simulink model "gm_uz_endat_interface_2025b"  (R2025b)
settings: Solver=FixedStepDiscrete  StartTime=0.0  StopTime=1.3e-3  RelTol=1e-3
undefined symbols (not defined in the file or in its folder): binary_or_gray, bit_sum, delay_first_clk_on_off, endat_clk_divider, endat_encoder_bit_width_multi_turn, endat_encoder_bit_width_single_turn, endat_encoder_number_of_CRC_bits, f_ADC, f_clock, PLL, t_ADC, t_clock, XData
libraries: hdlmdlgenlib x123, simulink x35, hdlsllib x29, simulink_extras x13
(part 4 of 4)

== system gm_uz_endat_interface_2025b/uz_endat_interface/position_to_speed_pll/Sine HDL Optimized/sincos hdl/cos_hdl ==
  note: (C) 2016 Mathworks, Inc
  In1 : Inport  OutDataTypeStr=fixdt(1, 27, 20)  SampleTime=1e-08
  1st or 4th Quad : Logic  Operator=OR  AllPortsSameDT=off  OutDataTypeStr=boolean  SampleTime=1e-08
  Amp25 : Sum  Inputs=+-  OutDataTypeStr=fixdt(1, 28, 27)  AccumDataTypeStr=fixdt(1, 28, 27)  SampleTime=1e-08
  Amp75 : Sum  Inputs=+-  OutDataTypeStr=fixdt(1, 28, 27)  AccumDataTypeStr=fixdt(1, 28, 27)  SampleTime=1e-08
  CastU16En1 : DataTypeConversion  OutDataTypeStr=fixdt(0, 10, 0)  ConvertRealWorld=Stored Integer (SI)  SampleTime=1e-08  SaturateOnIntegerOverflow=off  RndMeth=Floor
  CastU16En2 : DataTypeConversion  OutDataTypeStr=fixdt(0, 10, 0)  ConvertRealWorld=Stored Integer (SI)  SampleTime=1e-08  RndMeth=Floor
  CastU16En3 : DataTypeConversion  OutDataTypeStr=fixdt(0, 11, 0)  SampleTime=1e-08  SaturateOnIntegerOverflow=off  RndMeth=Floor
  GTEp75 : RelationalOperator  OutDataTypeStr=boolean  SampleTime=1e-08  InputSameDT=off
  LTEp25 : RelationalOperator  Operator=<=  OutDataTypeStr=boolean  SampleTime=1e-08  InputSameDT=off
  LTEp50 : RelationalOperator  Operator=<=  OutDataTypeStr=boolean  SampleTime=1e-08  InputSameDT=off
  Look-Up Table : Lookup_n-D  NumberOfTableDimensions=1  LookupTableObject=''  BreakpointsSpecification=Even spacing  BreakpointsForDimension1=XData  BreakpointsForDimension1FirstPoint=fi(0,0,InputWordLength,0)  BreakpointsForDimension1Spacing=fi(1,0,InputWordLength,0)  IndexSearchMethod=Evenly spaced points  Table=fi(YData,0, TableWordLength, TableFracLength)  TableDataTypeStr=fixdt(0, TableWordLength, TableFracLength)  InterpMethod=Flat  ExtrapMethod=Clip  OutDataTypeStr=fixdt(1,OutputWordLength,OutputFracLength)  LockScale=on
  Negate : UnaryMinus  SampleTime=1e-08
  Point25 : Constant  Value=0.25  OutDataTypeStr=fixdt(0, 27, 27)  SampleTime=1e-08
  Point50 : Constant  Value=0.5  OutDataTypeStr=fixdt(0, 27, 27)  SampleTime=1e-08
  Point75 : Constant  Value=0.75  OutDataTypeStr=fixdt(0, 27, 27)  SampleTime=1e-08
  Positive : DataTypeConversion  OutDataTypeStr=fixdt('sfix27_En20')
  QuadHandle1a : Switch  Criteria=u2 ~= 0  Threshold="fi(0,0,1,0,\"hex\",\"0\")"  OutDataTypeStr=fixdt(1, 28, 27)  SampleTime=1e-08  SaturateOnIntegerOverflow=off  InputSameDT=off
  QuadHandle1b : Switch  Criteria=u2 ~= 0  Threshold="fi(0,0,1,0,\"hex\",\"0\")"  OutDataTypeStr=fixdt(1, 28, 27)  SampleTime=1e-08  SaturateOnIntegerOverflow=off  InputSameDT=off
  QuadHandle2 : Switch  Criteria=u2 ~= 0  Threshold="fi(0,0,1,0,\"hex\",\"0\")"  OutDataTypeStr=fixdt(0, 10, 10)  SampleTime=1e-08  InputSameDT=off
  RAMDelayBalance : hdlmdlgenlib/Buffer
  Saturation : Saturate  UpperLimit="fi(0,0,10,0,\"hex\",\"0ff\")"  LowerLimit="fi(0,0,10,0,\"hex\",\"000\")"  SampleTime=1e-08  OutDataTypeStr=fixdt(0, 10, 0)
  SignCorrected : Switch  Criteria=u2 ~= 0  Threshold="fi(0,0,8,0,\"hex\",\"00\")"  OutDataTypeStr=fixdt(1, 27, 20)  SampleTime=1e-08  SaturateOnIntegerOverflow=off  InputSameDT=off
  Switch : Switch  Criteria=u2 ~= 0  Threshold="fi(0,0,1,0,\"hex\",\"0\")"  OutDataTypeStr=fixdt(0, 10, 0)  SampleTime=1e-08  SaturateOnIntegerOverflow=off  InputSameDT=off
  dtc : DataTypeConversion  OutDataTypeStr=uint8  ConvertRealWorld=Stored Integer (SI)  SampleTime=1e-08  SaturateOnIntegerOverflow=off  RndMeth=Floor
  insig : DataTypeConversion  OutDataTypeStr=fixdt(0, 10, 10)  SampleTime=1e-08  SaturateOnIntegerOverflow=off  RndMeth=Floor
  p25mA : Sum  Inputs=+-  OutDataTypeStr=fixdt(1, 28, 27)  AccumDataTypeStr=fixdt(1, 28, 27)  SampleTime=1e-08
  p75mA : Sum  Inputs=+-  OutDataTypeStr=fixdt(1, 28, 27)  AccumDataTypeStr=fixdt(1, 28, 27)  SampleTime=1e-08
  pow2switch : Constant  OutDataTypeStr=boolean  SampleTime=1e-08
  x : Outport  SampleTime=1e-08  VectorParamsAs1DForOutWhenUnconnected=off
  wires:
  LTEp25/1 -> 1st or 4th Quad/1, QuadHandle1a/2
  Point50/1 -> LTEp50/2
  In1/1 -> insig/1
  Point25/1 -> p25mA/1, Amp25/2, LTEp25/2
  insig/1 -> LTEp50/1, p25mA/2, GTEp75/1, Amp75/1, LTEp25/1, Amp25/1, p75mA/2
  Point75/1 -> p75mA/1, GTEp75/2, Amp75/2
  p25mA/1 -> QuadHandle1a/1
  GTEp75/1 -> QuadHandle1b/2, 1st or 4th Quad/2
  Amp25/1 -> QuadHandle1a/3
  LTEp50/1 -> QuadHandle2/2
  Amp75/1 -> QuadHandle1b/1
  p75mA/1 -> QuadHandle1b/3
  pow2switch/1 -> Switch/2
  1st or 4th Quad/1 -> dtc/1
  QuadHandle1a/1 -> QuadHandle2/1
  QuadHandle1b/1 -> QuadHandle2/3
  dtc/1 -> RAMDelayBalance/1
  RAMDelayBalance/1 -> SignCorrected/2
  QuadHandle2/1 -> CastU16En1/1
  CastU16En1/1 -> CastU16En3/1
  CastU16En3/1 -> CastU16En2/1
  CastU16En2/1 -> Switch/3, Saturation/1
  Saturation/1 -> Switch/1
  Switch/1 -> Look-Up Table/1
  Look-Up Table/1 -> Positive/1, Negate/1
  Positive/1 -> SignCorrected/1
  Negate/1 -> SignCorrected/3
  SignCorrected/1 -> x/1

== system gm_uz_endat_interface_2025b/uz_endat_interface/position_to_speed_pll/Sine HDL Optimized/sincos hdl/sin_hdl ==
  note: (C) 2016 Mathworks, Inc
  In1 : Inport  OutDataTypeStr=fixdt(1, 27, 20)  SampleTime=1e-08
  Amp50 : Sum  Inputs=+-  OutDataTypeStr=fixdt(1, 28, 27)  AccumDataTypeStr=fixdt(1, 28, 27)  SampleTime=1e-08
  CastU16En2 : DataTypeConversion  OutDataTypeStr=fixdt(0, 10, 0)  ConvertRealWorld=Stored Integer (SI)  SampleTime=1e-08  SaturateOnIntegerOverflow=off  RndMeth=Floor
  CastU16En3 : DataTypeConversion  OutDataTypeStr=fixdt(0, 10, 0)  ConvertRealWorld=Stored Integer (SI)  SampleTime=1e-08  RndMeth=Floor
  CastU16En4 : DataTypeConversion  OutDataTypeStr=fixdt(0, 11, 0)  SampleTime=1e-08  SaturateOnIntegerOverflow=off  RndMeth=Floor
  LTEp25 : RelationalOperator  Operator=<=  OutDataTypeStr=boolean  SampleTime=1e-08  InputSameDT=off
  LTEp50 : RelationalOperator  Operator=<=  OutDataTypeStr=boolean  SampleTime=1e-08  InputSameDT=off
  Look-Up Table : Lookup_n-D  NumberOfTableDimensions=1  LookupTableObject=''  BreakpointsSpecification=Even spacing  BreakpointsForDimension1=XData  BreakpointsForDimension1FirstPoint=fi(0,0,InputWordLength,0)  BreakpointsForDimension1Spacing=fi(1,0,InputWordLength,0)  IndexSearchMethod=Evenly spaced points  Table=fi(YData,0, TableWordLength, TableFracLength)  TableDataTypeStr=fixdt(0, TableWordLength, TableFracLength)  InterpMethod=Flat  ExtrapMethod=Clip  OutDataTypeStr=fixdt(1,OutputWordLength,OutputFracLength)  LockScale=on
  Negate : UnaryMinus  SampleTime=1e-08
  Point25 : Constant  Value=0.25  OutDataTypeStr=fixdt(0, 27, 27)  SampleTime=1e-08
  Point50 : Constant  Value=0.5  OutDataTypeStr=fixdt(0, 27, 27)  SampleTime=1e-08
  Positive : DataTypeConversion  OutDataTypeStr=fixdt('sfix27_En20')
  QuadHandle1 : Switch  Criteria=u2 ~= 0  Threshold="fi(0,0,1,0,\"hex\",\"0\")"  OutDataTypeStr=fixdt(1, 28, 27)  SampleTime=1e-08  SaturateOnIntegerOverflow=off  InputSameDT=off
  QuadHandle2 : Switch  Criteria=u2 ~= 0  Threshold="fi(0,0,1,0,\"hex\",\"0\")"  OutDataTypeStr=fixdt(0, 10, 10)  SampleTime=1e-08  SaturateOnIntegerOverflow=off  InputSameDT=off
  RAMDelayBalance : hdlmdlgenlib/Buffer
  Saturation : Saturate  UpperLimit="fi(0,0,10,0,\"hex\",\"0ff\")"  LowerLimit="fi(0,0,10,0,\"hex\",\"000\")"  SampleTime=1e-08  OutDataTypeStr=fixdt(0, 10, 0)
  SignCorrected : Switch  Criteria=u2 ~= 0  Threshold="fi(0,0,1,0,\"hex\",\"0\")"  OutDataTypeStr=fixdt(1, 27, 20)  SampleTime=1e-08  SaturateOnIntegerOverflow=off  InputSameDT=off
  Switch : Switch  Criteria=u2 ~= 0  Threshold="fi(0,0,1,0,\"hex\",\"0\")"  OutDataTypeStr=fixdt(0, 10, 0)  SampleTime=1e-08  SaturateOnIntegerOverflow=off  InputSameDT=off
  insig : DataTypeConversion  OutDataTypeStr=fixdt(0, 10, 10)  SampleTime=1e-08  SaturateOnIntegerOverflow=off  RndMeth=Floor
  p50mA : Sum  Inputs=+-  OutDataTypeStr=fixdt(1, 29, 27)  AccumDataTypeStr=fixdt(1, 29, 27)  SampleTime=1e-08
  pow2switch : Constant  OutDataTypeStr=boolean  SampleTime=1e-08
  y : Outport  SampleTime=1e-08  VectorParamsAs1DForOutWhenUnconnected=off
  wires:
  Negate/1 -> SignCorrected/3
  CastU16En3/1 -> Switch/3, Saturation/1
  Point50/1 -> p50mA/1, LTEp50/2, Amp50/2
  In1/1 -> insig/1
  LTEp25/1 -> QuadHandle2/2
  insig/1 -> QuadHandle1/1, LTEp50/1, Amp50/1
  LTEp50/1 -> QuadHandle1/2, RAMDelayBalance/1
  Amp50/1 -> QuadHandle1/3
  QuadHandle1/1 -> QuadHandle2/1, p50mA/2, LTEp25/1
  Point25/1 -> LTEp25/2
  p50mA/1 -> QuadHandle2/3
  RAMDelayBalance/1 -> SignCorrected/2
  QuadHandle2/1 -> CastU16En2/1
  CastU16En2/1 -> CastU16En4/1
  CastU16En4/1 -> CastU16En3/1
  Saturation/1 -> Switch/1
  pow2switch/1 -> Switch/2
  Switch/1 -> Look-Up Table/1
  Look-Up Table/1 -> Positive/1, Negate/1
  Positive/1 -> SignCorrected/1
  SignCorrected/1 -> y/1

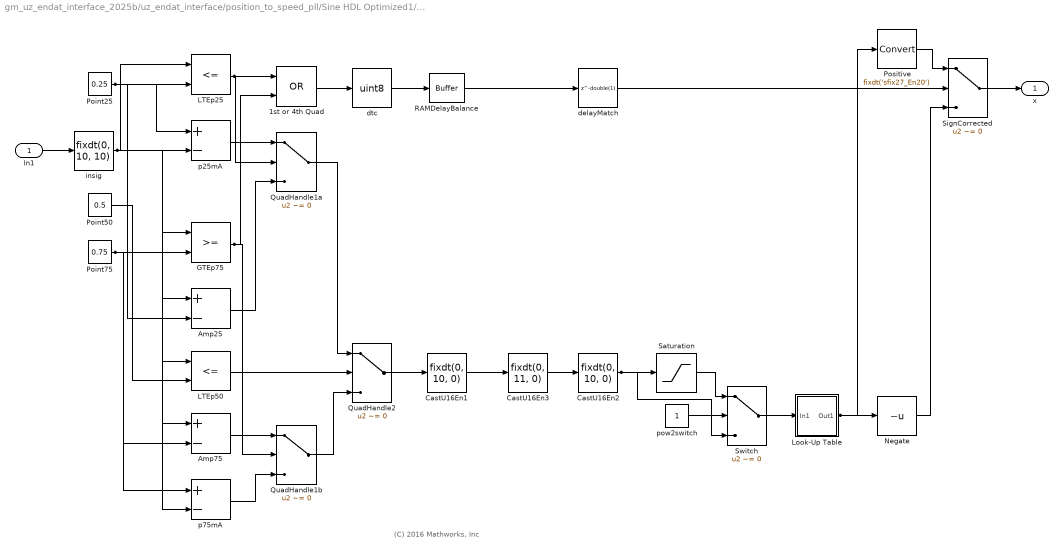
== system gm_uz_endat_interface_2025b/uz_endat_interface/position_to_speed_pll/Sine HDL Optimized1/sincos hdl/cos_hdl ==
  note: (C) 2016 Mathworks, Inc
  In1 : Inport  OutDataTypeStr=fixdt(1, 27, 20)  SampleTime=1e-08
  1st or 4th Quad : Logic  Operator=OR  AllPortsSameDT=off  OutDataTypeStr=boolean  SampleTime=1e-08
  Amp25 : Sum  Inputs=+-  OutDataTypeStr=fixdt(1, 28, 27)  AccumDataTypeStr=fixdt(1, 28, 27)  SampleTime=1e-08
  Amp75 : Sum  Inputs=+-  OutDataTypeStr=fixdt(1, 28, 27)  AccumDataTypeStr=fixdt(1, 28, 27)  SampleTime=1e-08
  CastU16En1 : DataTypeConversion  OutDataTypeStr=fixdt(0, 10, 0)  ConvertRealWorld=Stored Integer (SI)  SampleTime=1e-08  SaturateOnIntegerOverflow=off  RndMeth=Floor
  CastU16En2 : DataTypeConversion  OutDataTypeStr=fixdt(0, 10, 0)  ConvertRealWorld=Stored Integer (SI)  SampleTime=1e-08  RndMeth=Floor
  CastU16En3 : DataTypeConversion  OutDataTypeStr=fixdt(0, 11, 0)  SampleTime=1e-08  SaturateOnIntegerOverflow=off  RndMeth=Floor
  GTEp75 : RelationalOperator  OutDataTypeStr=boolean  SampleTime=1e-08  InputSameDT=off
  LTEp25 : RelationalOperator  Operator=<=  OutDataTypeStr=boolean  SampleTime=1e-08  InputSameDT=off
  LTEp50 : RelationalOperator  Operator=<=  OutDataTypeStr=boolean  SampleTime=1e-08  InputSameDT=off
  Look-Up Table : Subsystem
  Negate : UnaryMinus  SampleTime=1e-08
  Point25 : Constant  Value=0.25  OutDataTypeStr=fixdt(0, 27, 27)  SampleTime=1e-08
  Point50 : Constant  Value=0.5  OutDataTypeStr=fixdt(0, 27, 27)  SampleTime=1e-08
  Point75 : Constant  Value=0.75  OutDataTypeStr=fixdt(0, 27, 27)  SampleTime=1e-08
  Positive : DataTypeConversion  OutDataTypeStr=fixdt('sfix27_En20')
  QuadHandle1a : Switch  Criteria=u2 ~= 0  Threshold="fi(0,0,1,0,\"hex\",\"0\")"  OutDataTypeStr=fixdt(1, 28, 27)  SampleTime=1e-08  SaturateOnIntegerOverflow=off  InputSameDT=off
  QuadHandle1b : Switch  Criteria=u2 ~= 0  Threshold="fi(0,0,1,0,\"hex\",\"0\")"  OutDataTypeStr=fixdt(1, 28, 27)  SampleTime=1e-08  SaturateOnIntegerOverflow=off  InputSameDT=off
  QuadHandle2 : Switch  Criteria=u2 ~= 0  Threshold="fi(0,0,1,0,\"hex\",\"0\")"  OutDataTypeStr=fixdt(0, 10, 10)  SampleTime=1e-08  InputSameDT=off
  RAMDelayBalance : hdlmdlgenlib/Buffer
  Saturation : Saturate  UpperLimit="fi(0,0,10,0,\"hex\",\"0ff\")"  LowerLimit="fi(0,0,10,0,\"hex\",\"000\")"  SampleTime=1e-08  OutDataTypeStr=fixdt(0, 10, 0)
  SignCorrected : Switch  Criteria=u2 ~= 0  Threshold="fi(0,0,8,0,\"hex\",\"00\")"  OutDataTypeStr=fixdt(1, 27, 20)  SampleTime=1e-08  SaturateOnIntegerOverflow=off  InputSameDT=off
  Switch : Switch  Criteria=u2 ~= 0  Threshold="fi(0,0,1,0,\"hex\",\"0\")"  OutDataTypeStr=fixdt(0, 10, 0)  SampleTime=1e-08  SaturateOnIntegerOverflow=off  InputSameDT=off
  delayMatch : Delay  DelayLength=double(1)  InitialCondition=0
  dtc : DataTypeConversion  OutDataTypeStr=uint8  ConvertRealWorld=Stored Integer (SI)  SampleTime=1e-08  SaturateOnIntegerOverflow=off  RndMeth=Floor
  insig : DataTypeConversion  OutDataTypeStr=fixdt(0, 10, 10)  SampleTime=1e-08  SaturateOnIntegerOverflow=off  RndMeth=Floor
  p25mA : Sum  Inputs=+-  OutDataTypeStr=fixdt(1, 28, 27)  AccumDataTypeStr=fixdt(1, 28, 27)  SampleTime=1e-08
  p75mA : Sum  Inputs=+-  OutDataTypeStr=fixdt(1, 28, 27)  AccumDataTypeStr=fixdt(1, 28, 27)  SampleTime=1e-08
  pow2switch : Constant  OutDataTypeStr=boolean  SampleTime=1e-08
  x : Outport  SampleTime=1e-08  VectorParamsAs1DForOutWhenUnconnected=off
  wires:
  In1/1 -> insig/1
  LTEp25/1 -> QuadHandle1a/2, 1st or 4th Quad/1
  Point25/1 -> p25mA/1, LTEp25/2, Amp25/2
  insig/1 -> p75mA/2, LTEp50/1, p25mA/2, LTEp25/1, GTEp75/1, Amp75/1, Amp25/1
  GTEp75/1 -> QuadHandle1b/2, 1st or 4th Quad/2
  Point50/1 -> LTEp50/2
  Point75/1 -> p75mA/1, GTEp75/2, Amp75/2
  RAMDelayBalance/1 -> delayMatch/1
  p25mA/1 -> QuadHandle1a/1
  Amp25/1 -> QuadHandle1a/3
  Look-Up Table/1(Out1) -> Negate/1, Positive/1
  LTEp50/1 -> QuadHandle2/2
  Amp75/1 -> QuadHandle1b/1
  p75mA/1 -> QuadHandle1b/3
  1st or 4th Quad/1 -> dtc/1
  QuadHandle1a/1 -> QuadHandle2/1
  QuadHandle1b/1 -> QuadHandle2/3
  dtc/1 -> RAMDelayBalance/1
  QuadHandle2/1 -> CastU16En1/1
  CastU16En1/1 -> CastU16En3/1
  CastU16En3/1 -> CastU16En2/1
  delayMatch/1 -> SignCorrected/2
  CastU16En2/1 -> Switch/3, Saturation/1
  Saturation/1 -> Switch/1
  pow2switch/1 -> Switch/2
  Switch/1 -> Look-Up Table/1(In1)
  Positive/1 -> SignCorrected/1
  Negate/1 -> SignCorrected/3
  SignCorrected/1 -> x/1

== system gm_uz_endat_interface_2025b/uz_endat_interface/position_to_speed_pll/Sine HDL Optimized1/sincos hdl/sin_hdl ==
  note: (C) 2016 Mathworks, Inc
  In1 : Inport  OutDataTypeStr=fixdt(1, 27, 20)  SampleTime=1e-08
  Amp50 : Sum  Inputs=+-  OutDataTypeStr=fixdt(1, 28, 27)  AccumDataTypeStr=fixdt(1, 28, 27)  SampleTime=1e-08
  CastU16En2 : DataTypeConversion  OutDataTypeStr=fixdt(0, 10, 0)  ConvertRealWorld=Stored Integer (SI)  SampleTime=1e-08  SaturateOnIntegerOverflow=off  RndMeth=Floor
  CastU16En3 : DataTypeConversion  OutDataTypeStr=fixdt(0, 10, 0)  ConvertRealWorld=Stored Integer (SI)  SampleTime=1e-08  RndMeth=Floor
  CastU16En4 : DataTypeConversion  OutDataTypeStr=fixdt(0, 11, 0)  SampleTime=1e-08  SaturateOnIntegerOverflow=off  RndMeth=Floor
  LTEp25 : RelationalOperator  Operator=<=  OutDataTypeStr=boolean  SampleTime=1e-08  InputSameDT=off
  LTEp50 : RelationalOperator  Operator=<=  OutDataTypeStr=boolean  SampleTime=1e-08  InputSameDT=off
  Look-Up Table : Subsystem
  Negate : UnaryMinus  SampleTime=1e-08
  Point25 : Constant  Value=0.25  OutDataTypeStr=fixdt(0, 27, 27)  SampleTime=1e-08
  Point50 : Constant  Value=0.5  OutDataTypeStr=fixdt(0, 27, 27)  SampleTime=1e-08
  Positive : DataTypeConversion  OutDataTypeStr=fixdt('sfix27_En20')
  QuadHandle1 : Switch  Criteria=u2 ~= 0  Threshold="fi(0,0,1,0,\"hex\",\"0\")"  OutDataTypeStr=fixdt(1, 28, 27)  SampleTime=1e-08  SaturateOnIntegerOverflow=off  InputSameDT=off
  QuadHandle2 : Switch  Criteria=u2 ~= 0  Threshold="fi(0,0,1,0,\"hex\",\"0\")"  OutDataTypeStr=fixdt(0, 10, 10)  SampleTime=1e-08  SaturateOnIntegerOverflow=off  InputSameDT=off
  RAMDelayBalance : hdlmdlgenlib/Buffer
  Saturation : Saturate  UpperLimit="fi(0,0,10,0,\"hex\",\"0ff\")"  LowerLimit="fi(0,0,10,0,\"hex\",\"000\")"  SampleTime=1e-08  OutDataTypeStr=fixdt(0, 10, 0)
  SignCorrected : Switch  Criteria=u2 ~= 0  Threshold="fi(0,0,1,0,\"hex\",\"0\")"  OutDataTypeStr=fixdt(1, 27, 20)  SampleTime=1e-08  SaturateOnIntegerOverflow=off  InputSameDT=off
  Switch : Switch  Criteria=u2 ~= 0  Threshold="fi(0,0,1,0,\"hex\",\"0\")"  OutDataTypeStr=fixdt(0, 10, 0)  SampleTime=1e-08  SaturateOnIntegerOverflow=off  InputSameDT=off
  delayMatch : Delay  DelayLength=double(1)  InitialCondition=0
  insig : DataTypeConversion  OutDataTypeStr=fixdt(0, 10, 10)  SampleTime=1e-08  SaturateOnIntegerOverflow=off  RndMeth=Floor
  p50mA : Sum  Inputs=+-  OutDataTypeStr=fixdt(1, 29, 27)  AccumDataTypeStr=fixdt(1, 29, 27)  SampleTime=1e-08
  pow2switch : Constant  OutDataTypeStr=boolean  SampleTime=1e-08
  y : Outport  SampleTime=1e-08  VectorParamsAs1DForOutWhenUnconnected=off
  wires:
  Point50/1 -> p50mA/1, LTEp50/2, Amp50/2
  In1/1 -> insig/1
  LTEp50/1 -> QuadHandle1/2, RAMDelayBalance/1
  insig/1 -> QuadHandle1/1, LTEp50/1, Amp50/1
  QuadHandle1/1 -> QuadHandle2/1, p50mA/2, LTEp25/1
  pow2switch/1 -> Switch/2
  Saturation/1 -> Switch/1
  Amp50/1 -> QuadHandle1/3
  Point25/1 -> LTEp25/2
  RAMDelayBalance/1 -> delayMatch/1
  LTEp25/1 -> QuadHandle2/2
  p50mA/1 -> QuadHandle2/3
  delayMatch/1 -> SignCorrected/2
  QuadHandle2/1 -> CastU16En2/1
  CastU16En2/1 -> CastU16En4/1
  CastU16En4/1 -> CastU16En3/1
  CastU16En3/1 -> Switch/3, Saturation/1
  Switch/1 -> Look-Up Table/1(In1)
  Look-Up Table/1(Out1) -> Positive/1, Negate/1
  Negate/1 -> SignCorrected/3
  Positive/1 -> SignCorrected/1
  SignCorrected/1 -> y/1

== system gm_uz_endat_interface_2025b/uz_endat_interface/serial_communication/sample_serial_endat_data/Sample and Hold1/Model ==
  In : Inport  OutDataTypeStr=boolean  SampleTime=1e-08
  S : Inport  Port=2  OutDataTypeStr=boolean  SampleTime=1e-08
  Data Type Conversion : DataTypeConversion  OutDataTypeStr=boolean
  IC=ic : UnitDelay  SampleTime=1e-08
  Switch : Switch  Criteria=u2 ~= 0  Threshold="fi(0,0,1,0,\"hex\",\"0\")"  OutDataTypeStr=boolean  SampleTime=1e-08  InputSameDT=off
  Out : Outport  SampleTime=1e-08  InitialOutput=0
  wires:
  S/1 -> Data Type Conversion/1
  In/1 -> Switch/1
  Data Type Conversion/1 -> Switch/2
  IC=ic/1 -> Switch/3
  Switch/1 -> Out/1, IC=ic/1

== system gm_uz_endat_interface_2025b/uz_endat_interface/position_to_speed_pll/Sine HDL Optimized1/sincos hdl/cos_hdl/Look-Up Table ==
  In1 : Inport
  Look-Up Table : Lookup_n-D  NumberOfTableDimensions=1  LookupTableObject=''  BreakpointsSpecification=Even spacing  BreakpointsForDimension1=XData  BreakpointsForDimension1FirstPoint=fi(0,0,InputWordLength,0)  BreakpointsForDimension1Spacing=fi(1,0,InputWordLength,0)  IndexSearchMethod=Evenly spaced points  Table=fi(YData,0, TableWordLength, TableFracLength)  TableDataTypeStr=fixdt(0, TableWordLength, TableFracLength)  InterpMethod=Flat  ExtrapMethod=Clip  OutDataTypeStr=fixdt(1,OutputWordLength,OutputFracLength)  LockScale=on
  Look-Up Table_pd1 : Delay  DelayLength=1
  Out1 : Outport
  wires:
  In1/1 -> Look-Up Table/1
  Look-Up Table/1 -> Look-Up Table_pd1/1
  Look-Up Table_pd1/1 -> Out1/1

== system gm_uz_endat_interface_2025b/uz_endat_interface/position_to_speed_pll/Sine HDL Optimized1/sincos hdl/sin_hdl/Look-Up Table ==
  In1 : Inport
  Look-Up Table : Lookup_n-D  NumberOfTableDimensions=1  LookupTableObject=''  BreakpointsSpecification=Even spacing  BreakpointsForDimension1=XData  BreakpointsForDimension1FirstPoint=fi(0,0,InputWordLength,0)  BreakpointsForDimension1Spacing=fi(1,0,InputWordLength,0)  IndexSearchMethod=Evenly spaced points  Table=fi(YData,0, TableWordLength, TableFracLength)  TableDataTypeStr=fixdt(0, TableWordLength, TableFracLength)  InterpMethod=Flat  ExtrapMethod=Clip  OutDataTypeStr=fixdt(1,OutputWordLength,OutputFracLength)  LockScale=on
  Look-Up Table_pd1 : Delay  DelayLength=1
  Out1 : Outport
  wires:
  In1/1 -> Look-Up Table/1
  Look-Up Table_pd1/1 -> Out1/1
  Look-Up Table/1 -> Look-Up Table_pd1/1

== matlab function gm_uz_endat_interface_2025b/endat_encoder_Heidenhain_MT12bit_ST25bit/create_ST_and_MT_position_values/MATLAB Function ==
  data: u input; y output
function y = BinaryToGray(u)
%#codegen

y = bitxor(u,(bitshift(u,-1)));

== matlab function gm_uz_endat_interface_2025b/uz_endat_interface/wrap_2pi/fixed_point_floor/fixed_point_floor ==
  settings: fimath=fimath('RoundingMethod', 'Floor','OverflowAction', 'Wrap','ProductMode', 'FullPrecision', 'SumMode', 'FullPrecision')
  data: x input; y output
function y = fcn(x)
%#codegen
x_floor = bitsra(x, x.FractionLength);  % Shift right to remove fraction
x_floor = bitsll(x_floor, x.FractionLength);  % Shift left to restore scale

y = x_floor;

== matlab function gm_uz_endat_interface_2025b/uz_endat_interface/position_to_speed_pll/fixed_point_floor/fixed_point_floor ==
  settings: fimath=fimath('RoundingMethod', 'Floor','OverflowAction', 'Wrap','ProductMode', 'FullPrecision', 'SumMode', 'FullPrecision')
  data: x input; y output
function y = fcn(x)
%#codegen
x_floor = bitsra(x, x.FractionLength);  % Shift right to remove fraction
x_floor = bitsll(x_floor, x.FractionLength);  % Shift left to restore scale

y = x_floor;

== matlab function gm_uz_endat_interface_2025b/endat_encoder_Heidenhain_MT12bit_ST25bit/create_ST_and_MT_position_values/MATLAB Function1 ==
  data: u input; y output
function y = reverseBits(u)
%#codegen
% Reverse bit order for an unsigned fixed-point input (ufixN)

    % Determine word length from type
    BW = numerictype(u).WordLength;

    % Prepare output with same numerictype
    y = fi(0, numerictype(u), fimath(u));

    tmp = u;

    % Bit-by-bit reversal
    for i = 0:(BW-1)
        % Extract LSB, shift to MSB side, OR accumulate
        y = bitor(y, bitshift(bitand(tmp, fi(1, numerictype(u))), BW-1-i));
        tmp = bitshift(tmp, -1);
    end
end

== matlab function gm_uz_endat_interface_2025b/endat_encoder_Heidenhain_MT12bit_ST25bit/create_ST_and_MT_position_values/MATLAB Function2 ==
  data: u input; y output
function y = reverseBits(u)
%#codegen
% Reverse bit order for an unsigned fixed-point input (ufixN)

    % Determine word length from type
    BW = numerictype(u).WordLength;

    % Prepare output with same numerictype
    y = fi(0, numerictype(u), fimath(u));

    tmp = u;

    % Bit-by-bit reversal
    for i = 0:(BW-1)
        % Extract LSB, shift to MSB side, OR accumulate
        y = bitor(y, bitshift(bitand(tmp, fi(1, numerictype(u))), BW-1-i));
        tmp = bitshift(tmp, -1);
    end
end

== matlab function gm_uz_endat_interface_2025b/endat_encoder_Heidenhain_MT12bit_ST25bit/create_ST_and_MT_position_values/calc_crc ==
  data: clocks input; crc output; error1 input; error2 input; endat22 input; highpos input; lowpos input
function crc = MakeCrcPos(clocks, error1, error2, endat22, highpos, lowpos)
    % Initialize Flip-Flops
    ff = ones(1,5);  % 5 flip-flops set to 1
    code = zeros(1,66); % data bit array
    
    % Load alarm bits into code array
    if endat22
        code(1) = error1;
        code(2) = error2;
        startIdx = 1;
    else
        code(2) = error1;
        startIdx = 2;
    end
    
    % Load lowpos bits into code array
    for i = 3:34
        code(i) = bitand(lowpos, 1);
        lowpos = bitshift(lowpos, -1);
    end
    
    % Load highpos bits into code array
    for i = 35:66
        code(i) = bitand(highpos, 1);
        highpos = bitshift(highpos, -1);
    end
    
    % CRC calculation
    for i = startIdx:(clocks+2)  % adjust because MATLAB 1-based
        ex = xor(ff(5), code(i));
        ff_new = ff;
        ff_new(5) = ff(4);
        ff_new(4) = xor(ff(3), ex);
        ff_new(3) = ff(2);
        ff_new(2) = xor(ff(1), ex);
        ff_new(1) = ex;
        ff = ff_new;
    end
    
    % Store CRC in variable
    crc_tmp = 0;
    for i = 5:-1:1
        bitVal = ~ff(i);
        crc_tmp = bitshift(crc_tmp,1);
        crc_tmp = bitor(crc_tmp, bitVal);
    end
    crc=crc_tmp;
end

== matlab function gm_uz_endat_interface_2025b/endat_encoder_Heidenhain_MT12bit_ST25bit/MATLAB Function4 ==
  data: u input; y output; cnt input
function y = fcn(u,cnt)
%#codegen
tmp = bitget(u,cnt+1);
y = tmp;

== matlab function gm_uz_endat_interface_2025b/endat_encoder_Heidenhain_MT12bit_ST25bit/create_ST_and_MT_position_values/MATLAB Function3 ==
  data: u input; y output
function y = reverseBits(u)
%#codegen
% Reverse bit order for an unsigned fixed-point input (ufixN)

    % Determine word length from type
    BW = numerictype(u).WordLength;

    % Prepare output with same numerictype
    y = fi(0, numerictype(u), fimath(u));

    tmp = u;

    % Bit-by-bit reversal
    for i = 0:(BW-1)
        % Extract LSB, shift to MSB side, OR accumulate
        y = bitor(y, bitshift(bitand(tmp, fi(1, numerictype(u))), BW-1-i));
        tmp = bitshift(tmp, -1);
    end
end

== matlab function gm_uz_endat_interface_2025b/uz_endat_interface/serial_communication/MATLAB Function1/MATLAB Function1 ==
  data: clocks input; crc output; error1 input; error2 input; endat22 input; highpos input; lowpos input
function crc = MakeCrcPos(clocks, error1, error2, endat22, highpos, lowpos)
    % Initialize Flip-Flops
    ff = fi(ones(1,5),0,5,0);  % 5 flip-flops set to 1
    code = fi(zeros(1,64),0,64,0); % data bit array
    i = int32(0);

    
    % Load alarm bits into code array
    % if endat22
    %     code(1) = error1;
    %     code(2) = error2;
    %     startIdx = int32(1);
    % else
    %     code(2) = error1;
    %     startIdx = int32(2);
    % end
    
    % Load lowpos bits into code array
    for i = int32(3):int32(34)
        code(i) = bitand(lowpos, 1);
        lowpos = bitshift(lowpos, -1);
    end
    
    % Load highpos bits into code array
    for i = int32(35):int32(64)
        code(i) = bitand(highpos, 1);
        highpos = bitshift(highpos, -1);
    end
    
    % CRC calculation
    for i = int32(2):(int32(37)+int32(2))  % adjust because MATLAB 1-based
    % for i = startIdx:(clocks+int32(2))  % adjust because MATLAB 1-based
        ex = xor(ff(5), code(i));
        ff_new = ff;
        ff_new(5) = ff(4);
        ff_new(4) = xor(ff(3), ex);
        ff_new(3) = ff(2);
        ff_new(2) = xor(ff(1), ex);
        ff_new(1) = ex;
        ff = fi(ff_new,0,5,0);
    end
    
    % Store CRC in variable
    crc = uint32(0);
    for i = int32(5):int32(-1):int32(1)
        bitVal = uint32(~ff(i));
        crc = bitshift(crc,1);
        crc = bitor(crc, bitVal);
    end
end
